simulink model "Zad_2_sch"  (R2022a)
settings: Solver=VariableStepAuto  StartTime=0.0  StopTime=1  RelTol=1e-3
values from neighbouring files (symbols this model uses):
  a21 = (1/(2*m))*x30^2*(FemP1/FemP2^2)*exp(-x10/FemP2)    [Zad_2.m]
  a23 = -(1/m)*x30*(FemP1/FemP2)*exp(-x10/FemP2)    [Zad_2.m]
  a31 = (1/f1)*exp(x10/f2)*(ki*u10+ci-x30)    [Zad_2.m]
  a33 = -(f2/f1)*exp(x10/f2)    [Zad_2.m]
  b31 = ki*(f2/f1)*exp(x10/f2)    [Zad_2.m]
  g = 9.81    [Zad_2.m]
  xd = d-bd    (= 0.01326)    [Zad_2.m]
settings Model: Creator=marci  LastModifiedBy=marci

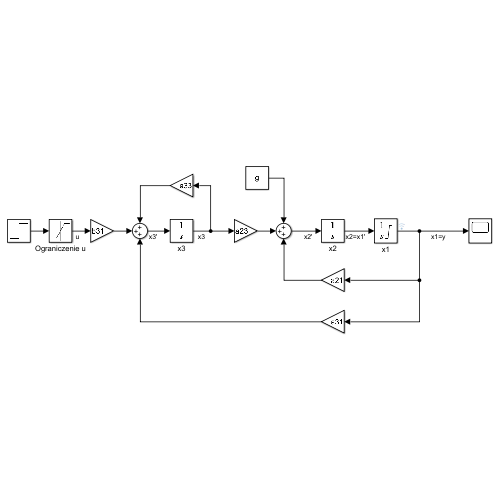
[thumbnail: Simulink's stored preview of the top-level diagram]
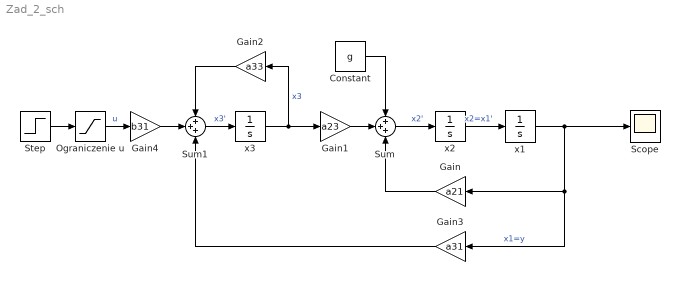
== system Zad_2_sch ==
  Constant : Constant  Value=g
  Gain : Gain  Gain=a21
  Gain1 : Gain  Gain=a23
  Gain2 : Gain  Gain=a33
  Gain3 : Gain  Gain=a31
  Gain4 : Gain  Gain=b31
  Ograniczenie u : Saturate  UpperLimit=1  LowerLimit=0
  Scope : Scope
  Step : Step  Time=0  SampleTime=0
  Sum : Sum  Inputs=+++
  Sum1 : Sum  Inputs=+++
  x1 : Integrator  InitialCondition=xd  LimitOutput=on  UpperSaturationLimit=xd  LowerSaturationLimit=0
  x2 : Integrator
  x3 : Integrator
  wires:
  x2/1 -> x1/1  "x2=x1'"
  x3/1 -> Gain1/1, Gain2/1  "x3"
  Sum/1 -> x2/1  "x2'"
  Sum1/1 -> x3/1  "x3'"
  Ograniczenie u/1 -> Gain4/1  "u"
  Step/1 -> Ograniczenie u/1
  Gain1/1 -> Sum/2
  Gain/1 -> Sum/3
  Constant/1 -> Sum/1
  Gain2/1 -> Sum1/1
  Gain3/1 -> Sum1/3
  Gain4/1 -> Sum1/2
  x1/1 -> Scope/1, Gain/1, Gain3/1  "x1=y"
